simulink model "example_PropRuleCast"  (R2019b)
settings: Solver=FixedStepDiscrete  StartTime=0.0  StopTime=0.9985  FixedStep=0.001  RelTol=1e-3  AbsTol=1e-6
libraries: fixpt_dtprop x2, DataTypePropCastLib x1
Description:
  | Fixed-Point to Fixed-Point Conversion
  | 
  | This example shows how to convert from one fixed-point data type to another fixed-point data type.
  | In this case the conversion is between sfix32_En2 and ufix8_En1, meaning:
  | 
  | * a signed 32-bit quantity with 2 bits to the right of the binary point
  | * an unsigned 8-bit quantity with 1 bit to the right of the binary point
settings Model: MinMaxOverflowLogging=MinMaxAndOverflow  ExtModeTrigMode=oneshot  ExtModeArmWhenConnect=off  ExtModeAutoUpdateStatusClock=off  Creator=The MathWorks, Inc.  LastModifiedBy=andyb
settings SolverCC: AutoScaleAbsTol=off
settings DataIOCC: SaveFormat=Array  ReturnWorkspaceOutputs=off  SignalLoggingName=sigsOut
settings OptimizationCC: BooleanDataType=off  ExpressionDepthLimit=2147483647  InitFltsAndDblsToZero=on  LifeSpan=inf
settings DebuggingCC: SaveWithParameterizedLinksMsg=none  UnderspecifiedInitializationDetection=Classic  MergeDetectMultiDrivingBlocksExec=none  SignalResolutionControl=TryResolveAllWithWarning  MultiTaskDSMMsg=warning  MultiTaskCondExecSysMsg=none  IntegerOverflowMsg=none  ParameterDowncastMsg=warning  ParameterOverflowMsg=warning  ParameterPrecisionLossMsg=none  FcnCallInpInsideContextMsg=warning  StateNameClashWarn=warning  SFUnexpectedBacktrackingDiag=warning  SFNoUnconditionalDefaultTransitionDiag=warning  SFExecutionAtInitializationDiag=none  IntegerSaturationMsg=none  ArithmeticOperatorsInVariantConditions=warning
settings HardwareCC: ProdBitPerPointer=32  ProdBitPerSizeT=32  ProdBitPerPtrDiffT=32  ProdLargestAtomicFloat=None  ProdIntDivRoundTo=Undefined  ProdEndianess=Unspecified  ProdWordSize=32  ProdHWDeviceType=ASIC/FPGA->ASIC/FPGA  TargetBitPerPointer=64  TargetBitPerSizeT=64  TargetBitPerPtrDiffT=64  TargetLongLongMode=on  TargetIntDivRoundTo=Zero  TargetEndianess=LittleEndian  TargetWordSize=64  TargetHWDeviceType=Custom Processor->MATLAB Host Computer  TargetUnknown=on  ProdEqTarget=off
settings ModelReferenceCC: PropagateSignalLabelsOutOfModel=off
settings SFSimCC: SimUseLocalCustomCode=off  CustomCodeUndefinedFunction=UseInterfaceOnly
settings RTWCC: RTWUseLocalCustomCode=off
settings CodeAppCC: StateflowObjectComments=on
settings GRTTargetCC: TargetFcnLib=ansi_tfl_tmw.mat  TargetLangStandard=C89/C90 (ANSI)  CombineOutputUpdateFcns=off  GRTInterface=on
settings ConfigComp: CovMetricSettings=d  CovHtmlReporting=on  CovSaveCumulativeToWorkspaceVar=on  CovSaveSingleToWorkspaceVar=on  CovExternalEMLEnable=off

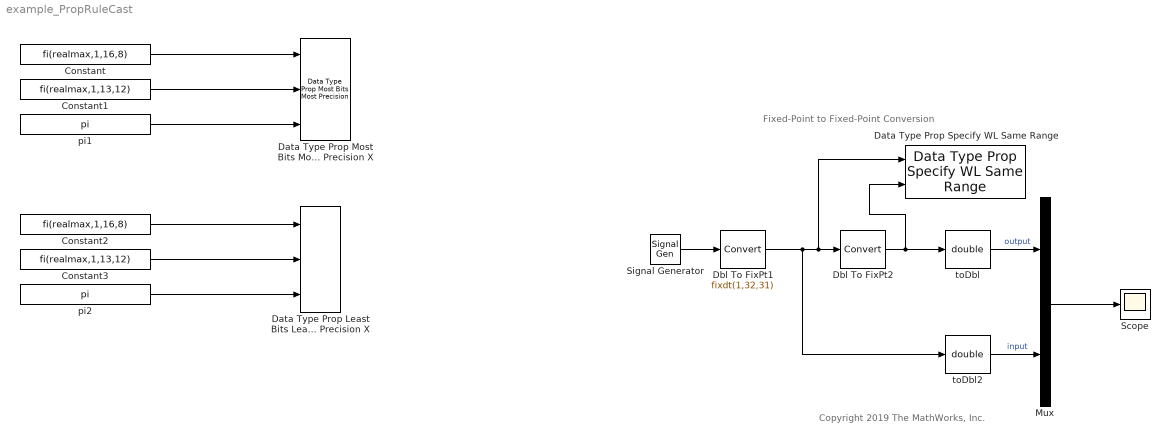
== system example_PropRuleCast ==
  note: Copyright 2019 The MathWorks, Inc.
  note: Fixed-Point to Fixed-Point Conversion
  Constant : Constant  Value=fi(realmax,1,16,8)
  Constant1 : Constant  Value=fi(realmax,1,13,12)
  Constant2 : Constant  Value=fi(realmax,1,16,8)
  Constant3 : Constant  Value=fi(realmax,1,13,12)
  Data Type Prop Least Bits Least Precision X : fixpt_dtprop/Data Type Prop Least Bits Least Precision  SystemSampleTime=-1  Latency=0  AutoFrameSizeCalculation=off
      settings: SourceProductName=Simulink  SourceProductBaseCode=SL
  Data Type Prop Most Bits Most Precision X : fixpt_dtprop/Data Type Prop Most Bits Most Precision  SystemSampleTime=-1  Latency=0  AutoFrameSizeCalculation=off
      settings: SourceProductName=Simulink  SourceProductBaseCode=SL
  Data Type Prop Specify WL Same Range : DataTypePropCastLib/DataType PropRules/Data Type Prop  Specify WL  Same Range  WLParam=4
  Dbl To FixPt1 : DataTypeConversion  OutDataTypeStr=fixdt(1,32,31)  RndMeth=Nearest  SaturateOnIntegerOverflow=on
  Dbl To FixPt2 : DataTypeConversion  RndMeth=Simplest  SaturateOnIntegerOverflow=on
  Mux : Mux  Inputs=2
  Scope : Scope
  Signal Generator : SignalGenerator  WaveForm=sawtooth  Amplitude=-1
  pi1 : Constant  Value=pi  OutDataTypeStr=Inherit: Inherit via back propagation
  pi2 : Constant  Value=pi  OutDataTypeStr=Inherit: Inherit via back propagation
  toDbl : DataTypeConversion  OutDataTypeStr=double
  toDbl2 : DataTypeConversion  OutDataTypeStr=double
  wires:
  Signal Generator/1 -> Dbl To FixPt1/1
  toDbl/1 -> Mux/1  "output"
  Dbl To FixPt1/1 -> Data Type Prop Specify WL Same Range/1, Dbl To FixPt2/1, toDbl2/1
  Mux/1 -> Scope/1
  Dbl To FixPt2/1 -> Data Type Prop Specify WL Same Range/2, toDbl/1
  toDbl2/1 -> Mux/2  "input"
  Constant/1 -> Data Type Prop Most Bits Most Precision X/1
  Constant1/1 -> Data Type Prop Most Bits Most Precision X/2
  pi1/1 -> Data Type Prop Most Bits Most Precision X/3
  pi2/1 -> Data Type Prop Least Bits Least Precision X/3
  Constant3/1 -> Data Type Prop Least Bits Least Precision X/2
  Constant2/1 -> Data Type Prop Least Bits Least Precision X/1
